simulink model "validazione_no_obs"  (R2023b)
settings: Solver=VariableStepAuto  StartTime=0.0  StopTime=T_end  RelTol=1e-3
values from neighbouring files (symbols this model uses):
  Ken_eta = K(:, 4)    [frequency_val_LQ_obsv1.m]    (also in frequency_val_LQ_obsv2.m; frequency_val_PP_no_obs.m = Ken(:, n+1:end); frequency_val_PP_obsv1.m = Ken(:, n+1:end); frequency_val_PP_obsv2.m = Ken(:, n+1:end))
  Ken_x = K(:, 1:3)    [frequency_val_LQ_obsv1.m]    (also in frequency_val_LQ_obsv2.m; frequency_val_PP_no_obs.m = Ken(:, 1:n); frequency_val_PP_obsv1.m = Ken(:, 1:n); frequency_val_PP_obsv2.m = Ken(:, 1:n))
undefined symbols (not defined in the file or in its folder): Lc, Rtot, x1_eq0, x2_eq0, x3_eq0
libraries: simulink x1
settings Model: Creator=Pronto all'uso  LastModifiedBy=Pronto all'uso
settings SolverCC: AlgebraicLoopSolver=TrustRegion

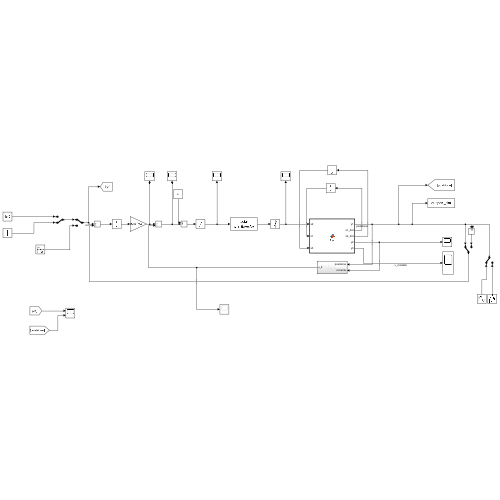
[thumbnail: Simulink's stored preview of the top-level diagram]
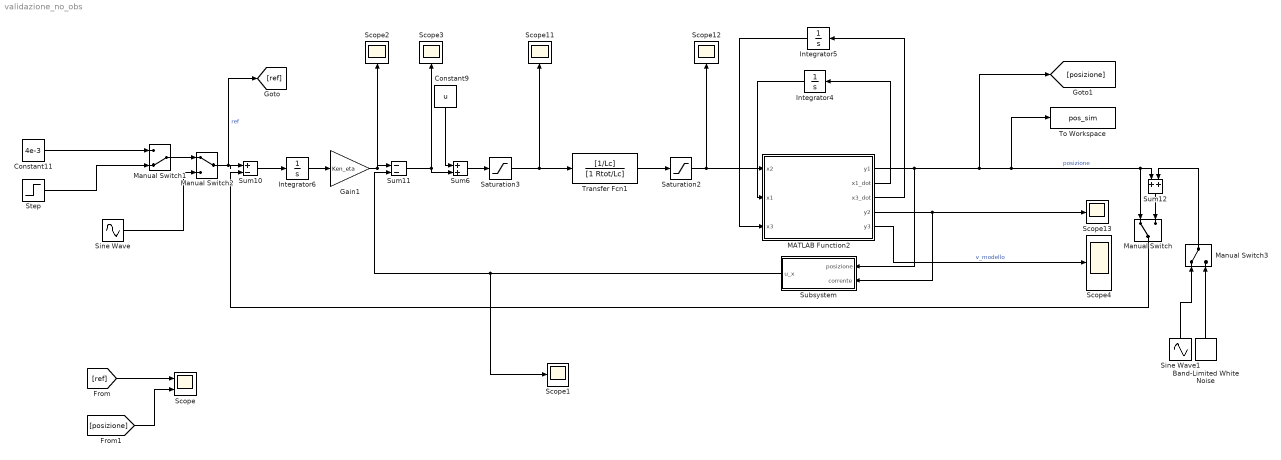
== system validazione_no_obs ==
  Band-Limited White Noise : simulink/Sources/Band-Limited White Noise  Cov=[8.9934e-11*0.002]  Ts=0.002  seed=[23341]
  Constant11 : Constant  Value=4e-3
  Constant9 : Constant  Value=u
  Gain1 : Gain  Gain=Ken_eta  SaturateOnIntegerOverflow=on  OutDataTypeStr=Inherit: Same as input  ParamDataTypeStr=Inherit: Same as input
  Integrator4 : Integrator
  Integrator5 : Integrator
  Integrator6 : Integrator
  MATLAB Function2 : MATLAB Function  TreatAsAtomicUnit=on
  Manual Switch : ManualSwitch
  Manual Switch1 : ManualSwitch  CurrentSetting=0
  Manual Switch2 : ManualSwitch
  Manual Switch3 : ManualSwitch
  Saturation2 : Saturate  UpperLimit=3  LowerLimit=0
  Saturation3 : Saturate  UpperLimit=23  LowerLimit=0
  Scope : Scope  NumInputPorts=2
  Scope{1..4,11..13} (7 alike) : Scope
  Sine Wave : Sin  Amplitude=0.001  Bias=0.004  Frequency=4  SampleTime=0
  Sine Wave1 : Sin  Amplitude=0.00001  Frequency=50  SampleTime=0.002
  Step : Step  Time=2  After=0.004  SampleTime=0.002
  Subsystem : Subsystem
  Sum10 : Sum  Inputs=|+-  InputSameDT=on  SaturateOnIntegerOverflow=on  OutDataTypeStr=Inherit: Same as first input
  Sum11 : Sum  Inputs=|--  InputSameDT=on  SaturateOnIntegerOverflow=on  OutDataTypeStr=Inherit: Same as first input
  Sum12 : Sum  Inputs=|++  InputSameDT=on  SaturateOnIntegerOverflow=on  OutDataTypeStr=Inherit: Same as first input
  Sum6 : Sum  Inputs=++|  InputSameDT=on  SaturateOnIntegerOverflow=on  OutDataTypeStr=Inherit: Same as first input
  To Workspace : ToWorkspace  VariableName=pos_sim  SampleTime=0.002
  Transfer Fcn1 : TransferFcn  Numerator=[1/Lc]  Denominator=[1 Rtot/Lc]
  wires:
  Integrator5/1 -> MATLAB Function2/3(x3)
  MATLAB Function2/3(x3_dot) -> Integrator5/1
  Transfer Fcn1/1 -> Saturation2/1
  Sum11/1 -> Scope3/1, Sum6/2
  Integrator6/1 -> Gain1/1
  Manual Switch3/1 -> Sum12/2
  Saturation2/1 -> MATLAB Function2/1(x2), Scope12/1
  Manual Switch1/1 -> Manual Switch2/1
  Sum6/1 -> Saturation3/1
  MATLAB Function2/1(y1) -> Subsystem/1(posizione), [posizione], To Workspace/1, Sum12/1, Manual Switch/1  "posizione"
  Sum12/1 -> Manual Switch/2
  Integrator4/1 -> MATLAB Function2/2(x1)
  Sine Wave/1 -> Manual Switch2/2
  MATLAB Function2/4(y2) -> Subsystem/2(corrente), Scope13/1
  Manual Switch2/1 -> [ref], Sum10/1  "ref"
  Constant9/1 -> Sum6/1
  Gain1/1 -> Sum11/1, Scope2/1
  Sine Wave1/1 -> Manual Switch3/1
  MATLAB Function2/2(x1_dot) -> Integrator4/1
  Sum10/1 -> Integrator6/1
  Saturation3/1 -> Transfer Fcn1/1, Scope11/1
  MATLAB Function2/5(y3) -> Scope4/1  "v_modello"
  Subsystem/1(u_x) -> Sum11/2, Scope1/1
  [ref] -> Scope/1
  [posizione] -> Scope/2
  Constant11/1 -> Manual Switch1/1
  Step/1 -> Manual Switch1/2
  Band-Limited White Noise/1 -> Manual Switch3/2
  Manual Switch/1 -> Sum10/2

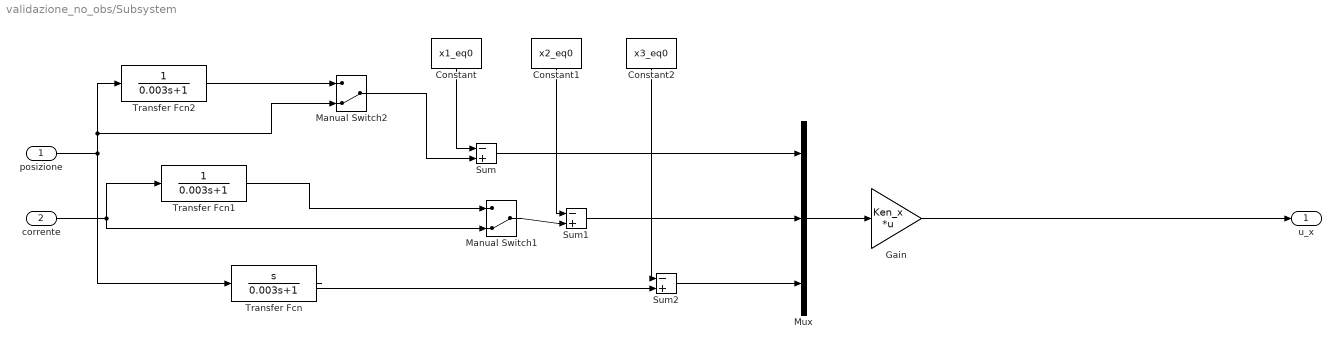
== system validazione_no_obs/Subsystem ==
  posizione : Inport
  corrente : Inport  Port=2
  Constant : Constant  Value=x1_eq0
  Constant1 : Constant  Value=x2_eq0
  Constant2 : Constant  Value=x3_eq0
  Gain : Gain  Gain=Ken_x  Multiplication=Matrix(K*u) (u vector)  SaturateOnIntegerOverflow=on  OutDataTypeStr=Inherit: Same as input  ParamDataTypeStr=Inherit: Same as input
  Manual Switch1 : ManualSwitch  CurrentSetting=0
  Manual Switch2 : ManualSwitch  CurrentSetting=0
  Mux : Mux  Inputs=3
  Sum : Sum  Inputs=-+|  InputSameDT=on  SaturateOnIntegerOverflow=on  OutDataTypeStr=Inherit: Same as first input
  Sum1 : Sum  Inputs=-+|  InputSameDT=on  SaturateOnIntegerOverflow=on  OutDataTypeStr=Inherit: Same as first input
  Sum2 : Sum  Inputs=-+|  InputSameDT=on  SaturateOnIntegerOverflow=on  OutDataTypeStr=Inherit: Same as first input
  Transfer Fcn : TransferFcn  Numerator=[1 0]  Denominator=[0.003 1]
  Transfer Fcn1 : TransferFcn  Denominator=[0.003 1]
  Transfer Fcn2 : TransferFcn  Numerator=[1 ]  Denominator=[0.003 1]
  u_x : Outport
  wires:
  Constant/1 -> Sum/1
  Constant1/1 -> Sum1/1
  Constant2/1 -> Sum2/1
  Sum/1 -> Mux/1
  Sum2/1 -> Mux/3
  Sum1/1 -> Mux/2
  Mux/1 -> Gain/1
  Gain/1 -> u_x/1
  Transfer Fcn/1 -> Sum2/2
  posizione/1 -> Manual Switch2/2, Transfer Fcn2/1, Transfer Fcn/1
  corrente/1 -> Manual Switch1/2, Transfer Fcn1/1
  Transfer Fcn1/1 -> Manual Switch1/1
  Manual Switch1/1 -> Sum1/2
  Transfer Fcn2/1 -> Manual Switch2/1
  Manual Switch2/1 -> Sum/2

== matlab function validazione_no_obs/MATLAB Function2 ==
  data: y1 output; x2 input; x1_dot output; x1 input; x3 input; x3_dot output; y2 output; y3 output
function [y1,x1_dot, x3_dot, y2, y3] = fcn(x2, x1, x3)
    m = 0.0657;
    g = 9.81;
    k_mag = 2.4405e-05;
    Rtot = 9.7585;
    Lc = 0.3708;
    y0 = 0.012;
    
    x1_dot = x3;
    x3_dot = (k_mag/m)*(x2/(y0-x1))^2 - g;

    if x1 <= 0 && x3_dot < 0
        x1 = 0;
        x3 = 0;
        x3_dot = 0;
    end
y1 = x1;
y2 = x2;
y3 = x3;
